simulink model "model"  (R2020b)
settings: Solver=VariableStepAuto  StartTime=0.0  StopTime=tStop  MaxStep=0.01  RelTol=1e-3
values from neighbouring files (symbols this model uses):
  b = 50    [init.m]
  k1 = 50    [init.m]
  k12 = 100    [init.m]
  m1 = 100    [init.m]
  m2 = 200    [init.m]
settings Model: Creator=Admin  LastModifiedBy=Admin
settings DataIOCC: ExternalInput=[t, F]  LoadExternalInput=on  SaveFormat=Array

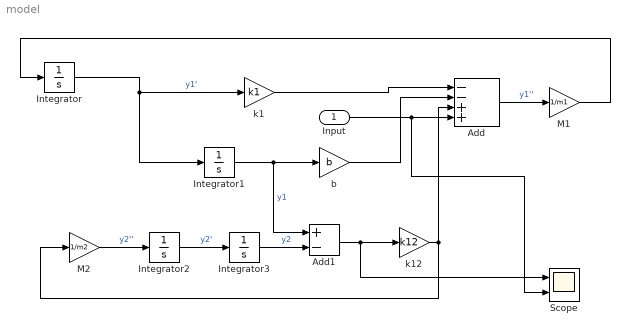
== system model ==
  Input : Inport
  Add : Sum  Inputs=--++
  Add1 : Sum  Inputs=+-
  Integrator{,1..3} (4 alike) : Integrator
  M1 : Gain  Gain=1/m1
  M2 : Gain  Gain=1/m2
  Scope : Scope  NumInputPorts=2
  b : Gain  Gain=b
  k1 : Gain  Gain=k1
  k12 : Gain  Gain=k12
  wires:
  M2/1 -> Integrator2/1  "y2''"
  Integrator/1 -> Integrator1/1, k1/1  "y1'"
  k1/1 -> Add/1
  M1/1 -> Integrator/1
  Integrator1/1 -> Add1/1, b/1  "y1"
  Input/1 -> Scope/2, Add/4
  Integrator2/1 -> Integrator3/1  "y2'"
  b/1 -> Add/2
  Integrator3/1 -> Add1/2  "y2"
  k12/1 -> M2/1, Add/3
  Add/1 -> M1/1  "y1''"
  Add1/1 -> Scope/1, k12/1
